simulink model "Citation_2015a"  (R2015a)
settings: Solver=ode5  StartTime=0.0  StopTime=inf  FixedStep=0.01  RelTol=1e-3
InitFcn:
  | initcit
values from neighbouring files (symbols this model uses):
  aeroinit = [dp_ini;inicoef('CX0');inicoef('CXa');inicoef('CXa2');inicoef('CXq')     ;inicoef('CXde');inicoef('CY0');inicoef('CYB');inicoef('CYp');inicoef('CYr')     ;inicoef('CYda');inicoef('CYdr');inicoef('CZ0');inicoef('CZa');inicoef('CZq')     ;inicoef('CZde');inicoef('Cl0');inicoef('ClB');inicoef('Clp');inicoef('Clr')     ;inicoef('Clda');inicoef('Cldr');inicoef('Cm0');inicoef('Cma');inicoef('Cmq')     ; ...(+113 chars)    [initcit.m]
  Clda_thresh = 3.410e-2/2    (= 0.01705)    [initcit.m]
  h_l_old = zeros(6,sample_size)    [initcit.m]
  h_m_old = zeros(4,sample_size)    [initcit.m]
  h_n_old = zeros(6,sample_size)    [initcit.m]
  h_X_old = zeros(5,sample_size)    [initcit.m]
  h_Y_old = zeros(6,sample_size)    [initcit.m]
  h_Z_old = zeros(4,sample_size)    [initcit.m]
  I = [massinit(5),0, -massinit(8);0, massinit(6),0;-massinit(8),0, massinit(7)]    [initcit.m]
  p_l = [inicoef('Cl0');inicoef('ClB');inicoef('Clp');inicoef('Clr')     ;inicoef('Clda');inicoef('Cldr')].*ones(6,sample_size)    [initcit.m]
  p_m = [inicoef('Cm0');inicoef('Cma');inicoef('Cmq')     ;inicoef('Cmde')].*ones(4,sample_size)    [initcit.m]
  p_n = [inicoef('Cn0');inicoef('CnB');inicoef('Cnp');inicoef('Cnr')     ;inicoef('Cnda');inicoef('Cndr')].*ones(6,sample_size)    [initcit.m]
  p_X = [inicoef('CX0');inicoef('CXa');inicoef('CXa2');inicoef('CXq')     ;inicoef('CXde')].*ones(5,sample_size)    [initcit.m]
  p_Y = [inicoef('CY0');inicoef('CYB');inicoef('CYp');inicoef('CYr')     ;inicoef('CYda');inicoef('CYdr')].*ones(6,sample_size)    [initcit.m]
  p_Z = [inicoef('CZ0');inicoef('CZa');inicoef('CZq')     ;inicoef('CZde')].*ones(4,sample_size)    [initcit.m]
  Pcov_l = 10000*eye(6)    [initcit.m]
  Pcov_m = 10000*eye(4)    [initcit.m]
  Pcov_n = 10000*eye(6)    [initcit.m]
  Pcov_X = 10000*eye(5)    [initcit.m]
  Pcov_Y = 10000*eye(6)    [initcit.m]
  Pcov_Z = 10000*eye(4)    [initcit.m]
  replay = 0    [initcit.m]
  T0 = 288.15    [rho_test.m]
  timeend = inputsim.data{1}.Values.Time(end)    [initcit.m]
  Vw915 = 0    [initcit.m]
  winddir = 45*(pi/180)    (= 0.785398163397)    [initcit.m]
  x0 = []    [cessnac550_3d_sfnc.m]    (also in sfunxyauto.m)
  y_l = zeros(1,sample_size)    [initcit.m]
  y_l_est_old = zeros(size(y_l))    [initcit.m]
  y_m = zeros(1,sample_size)    [initcit.m]
  y_m_est_old = zeros(size(y_m))    [initcit.m]
  y_n = zeros(1,sample_size)    [initcit.m]
  y_n_est_old = zeros(size(y_n))    [initcit.m]
  y_X = zeros(1,sample_size)    [initcit.m]
  y_X_est_old = zeros(size(y_X))    [initcit.m]
  y_Y = zeros(1,sample_size)    [initcit.m]
  y_Y_est_old = zeros(size(y_Y))    [initcit.m]
  y_Z = zeros(1,sample_size)    [initcit.m]
  y_Z_est_old = zeros(size(y_Z))    [initcit.m]
undefined symbols (not defined in the file or in its folder): chord, cv1, cv2, cv3, cv4, deltagmax1, deltagmax2, deltagmax3, deltagmax4, Deng, ealphag, ealphas, g0, hDME, hGS, kt1, kt2, kt3, lh, massinit, matbuaf, matdaf, matdam, matdbbf, matdeaf, matdgaf, matdqaf, matduaf, matdwaw, matedhr, mateif, matelhr, matemhr, matemv1, matemv2, matemve, matetam, mateuaf, matfaaf, matfaxl, matff, matibaf, matibmh, matipaf, matipmh, matiraf, matiuaf, matiwaf, matlaf, matlam, matleaf, matleam, matlgaf, matlqaf, matluaf, matmaaf, matmaam, matmaf, matmam, matmbbf ... (+74)
undefined symbols (not defined in the file): matibb
libraries: simulink x13, templibrary x6, vrlib x1
(part 2 of 7)

== system Citation_2015a/Aerodynamic Parameter Estimation/alternative failure monitor system ==
  note: this failure monitoring systems looks at the parameter related to the estimated delta_a directly. E.g. Clda
  In2 : Inport
  In3 : Inport  Port=2
  Abs : Abs
  Auto_correlation : Subsystem
  Constant : Constant  Value=Clda_thresh*2
  Constant4 : Constant
  Constant5 : Constant  Value=0
  Demux : Demux  Commented=on  Outputs=2
  Detect Change : simulink/Logic and Bit Operations/Detect Change  vinit=0  OutDataTypeStr=boolean
  Display : Display  Commented=on
  Failure Monitor : TimeScope  Commented=on  DefaultConfigurationName=spbscopes.TimeScopeBlockCfg  NumInputPorts=3
  Gain : Gain  Gain=0.5
  Memory : Memory
  Selector : Selector  NumberOfDimensions=2  InputPortWidth=1  IndexOptions=Index vector (dialog),Index vector (dialog)  Indices=[5],[1:50]  OutputSizes=1,1
  Send diagnostic message : Subsystem  Commented=on  TreatAsAtomicUnit=on
  Slider : Subsystem  Description=Replaced Block  mask(Replaced Block){}
      mask help: This block has been replaced with an empty subsystem because it used functionality that is unavailable in Simulink R2015a.
      mask Display: fprintf('Replaced: %s\n','Dashboard Widget')
  Sum : Sum  Inputs=|+-
  Switch : Switch  Criteria=u2 > Threshold  Threshold=Clda_thresh
  Variance : TimeScope  Commented=on  DefaultConfigurationName=spbscopes.TimeScopeBlockCfg  NumInputPorts=3
  auto corr : TimeScope  Commented=on  DefaultConfigurationName=spbscopes.TimeScopeBlockCfg  NumInputPorts=2
  moving average square : MATLAB Function  TreatAsAtomicUnit=on
      settings: PermitHierarchicalResolution=ParametersOnly
  variance : Subsystem  Commented=on
  Out1 : Outport
  wires:
  In3/1 -> Auto_correlation/2(kgap)
  Selector/1 -> Auto_correlation/1(delta_window), moving average square/1(delta)
  moving average square/1(av) -> Sum/1, Failure Monitor/3  "Alt Moving square average"
  variance/2(sigma_avg) -> Demux/1
  Sum/1 -> Abs/1
  Constant/1 -> Gain/1, Sum/2
  Demux/2 -> Variance/3
  variance/1(variance) -> Variance/1
  Demux/1 -> Variance/2
  In2/1 -> Selector/1
  Constant5/1 -> Switch/3
  Constant4/1 -> Switch/1
  Switch/1 -> Failure Monitor/1, Display/1, Memory/1  "alt failure detected"
  Auto_correlation/1(PI_kgap) -> auto corr/1
  Auto_correlation/2(PI_kgap_avg) -> auto corr/2
  Memory/1 -> Send diagnostic message/Trigger, Send diagnostic message/1(In1), Detect Change/1
  Gain/1 -> Failure Monitor/2  "alt threshold"
  Detect Change/1 -> Out1/1
  Abs/1 -> Switch/2

== system Citation_2015a/Aerodynamic Parameter Estimation/get_h_vectors ==
  input : Inport
  model output : Inport  Port=2
  1 : Terminator
  6 : Terminator
  Constant : Constant
  Constant1 : Constant  Value=chord
  Constant2 : Constant  Value=span
  Demux4 : Demux  Outputs=[1 1 1 1 1 1 31]
  Demux5 : Demux  Outputs=[1 1 1 7]
  Divide : Product  Inputs=*/
  Divide1 : Product  Inputs=*/
  Divide2 : Product  Inputs=*/
  Gain : Gain  Gain=2
  Multiply : Product
  Multiply1 : Product
  Mux : Mux  Inputs=6
  Mux1 : Mux  Inputs=5
  Mux2 : Mux
  Mux3 : Mux  Inputs=6
  Product : Product
  Product1 : Product
  hk : Outport
  wires:
  Demux5/2 -> Mux/5  "da"
  Demux4/6 -> Mux/2  "beta"
  Demux4/5 -> Mux1/2, Product/2, Mux2/2, Product/1  "alpha"
  Constant/1 -> Mux1/1, Mux/1, Mux2/1
  Demux4/3 -> Multiply1/1  "r"
  Demux5/4 -> 6/1
  Demux4/2 -> Product1/1  "q"
  Demux4/1 -> Multiply/2  "p"
  Demux4/4 -> Gain/1, Divide/2  "vtas"
  Constant1/1 -> Product1/2
  Product1/1 -> Divide/1
  Divide/1 -> Mux2/3, Mux1/4  "qc/V"
  model output/1 -> Demux4/1
  Demux5/1 -> Mux2/4, Mux1/5  "de"
  Product/1 -> Mux1/3
  Demux5/3 -> Mux/6  "dr"
  input/1 -> Demux5/1
  Mux1/1 -> Mux3/1  "hk_CX"
  Mux2/1 -> Mux3/3, Mux3/5  "hk_CZ & hk_Cm"
  Demux4/7 -> 1/1
  Constant2/1 -> Multiply1/2, Multiply/1
  Multiply/1 -> Divide1/1
  Gain/1 -> Divide2/2, Divide1/2
  Divide1/1 -> Mux/3  "pb/2V"
  Multiply1/1 -> Divide2/1
  Divide2/1 -> Mux/4  "rb/2V"
  Mux/1 -> Mux3/2, Mux3/6, Mux3/4
  Mux3/1 -> hk/1

== system Citation_2015a/Cessna Citation 500/Actuators ==
  note: Failure will not be visible here
  note: de
      | da
      | dr
      | dte
      | dta
      | dtr
      | df
      | gear
      | pla1
      | pla2
  note: de
      | da
      | dr
      | dte
      | dta
      | dtr
      | df
      | gear
      | pla1
      | pla2
  In : Inport
  "failure toggle " : Inport  Port=2
  Demux : Demux  Outputs=10
  Gain : Gain  Gain=0.5
  Mux : Mux  Inputs=10
  Mux2 : Mux  Inputs=10
  Subsystem : Subsystem  Commented=on
  Sum : Sum  Inputs=|++
  Switch : Switch  Criteria=u2 > Threshold
  Time Scope : TimeScope  Commented=on  DefaultConfigurationName=spbscopes.TimeScopeBlockCfg
  "aileron failure offset (deg) " : Constant  Value=16
  da : Subsystem
  da limits : Saturate  UpperLimit=0.65  LowerLimit=-0.65
  da limits1 : Saturate  UpperLimit=0.65  LowerLimit=-0.65
  da limits2 : Saturate  UpperLimit=0.65  LowerLimit=-0.65
  da2 : Subsystem
  de : Subsystem
  de limits : Saturate  UpperLimit=0.26  LowerLimit=-0.35
  deg2rad : Gain  Gain=pi/180
  dr : Subsystem
  dr limits : Saturate  UpperLimit=0.38  LowerLimit=-0.38
  flaps : Subsystem
  gear : Subsystem
  Actuator_True : Outport
  Actuator_pred : Outport  Port=2
  wires:
  In/1 -> Demux/1
  Mux/1 -> Actuator_True/1
  Demux/1 -> de/1(In)
  Demux/2 -> Switch/3, da limits1/1, da/1(In)  "da desired"
  Demux/3 -> dr/1(In)
  de/1(Out) -> de limits/1
  da/1(Out) -> da limits/1
  dr/1(Out) -> dr limits/1
  dr limits/1 -> Mux2/3, Mux/3
  de limits/1 -> Mux/1, Mux2/1
  Demux/8 -> gear/1(In)
  Demux/7 -> flaps/1(In)
  Demux/9 -> Mux2/9, Mux/9
  Demux/10 -> Mux2/10, Mux/10
  flaps/1(Out) -> Mux2/7, Mux/7
  gear/1(Out) -> Mux/8, Mux2/8
  Demux/4 -> Mux2/4, Mux/4
  Demux/5 -> Mux2/5, Mux/5
  Demux/6 -> Mux2/6, Mux/6
  da limits/1 -> Mux2/2
  "aileron failure offset (deg) "/1 -> deg2rad/1
  deg2rad/1 -> Sum/1  "da offset"
  Gain/1 -> Sum/2
  Switch/1 -> da2/1(In)
  Mux2/1 -> Actuator_pred/1
  "failure toggle "/1 -> Switch/2
  Sum/1 -> Switch/1
  da limits2/1 -> Time Scope/1, Mux/2
  da2/1(Out) -> da limits2/1
  da limits1/1 -> Gain/1

== system Citation_2015a/Cessna Citation 500/Citation model DASMAT ==
  ua : Inport
  ut : Inport  Port=2
  Environment : Inport  Port=3
  AIRCRAFT MODEL : Subsystem
  Mux1 : Mux  Inputs=[8 2 8 12 8]
  Terminator_{16..19} (4 alike) : Terminator
  massinit : Constant  Value=massinit
  x : Outport
  xdot : Outport  Port=2
  yair : Outport  Port=3
  yacc : Outport  Port=4
  yfp : Outport  Port=5
  ypp : Outport  Port=6
  wires:
  AIRCRAFT MODEL/13(FMt) -> Terminator_19/1
  Mux1/1 -> yair/1
  AIRCRAFT MODEL/12(FMag) -> Terminator_17/1
  AIRCRAFT MODEL/11(FMa) -> Terminator_18/1
  AIRCRAFT MODEL/7(gust) -> Mux1/5
  AIRCRAFT MODEL/6(wind) -> Mux1/4
  AIRCRAFT MODEL/5(yad2) -> Mux1/3
  AIRCRAFT MODEL/4(yad1) -> Mux1/2
  AIRCRAFT MODEL/3(yatm) -> Mux1/1
  AIRCRAFT MODEL/2(xdot) -> xdot/1
  AIRCRAFT MODEL/1(x) -> x/1
  AIRCRAFT MODEL/10(ys) -> Terminator_16/1
  AIRCRAFT MODEL/9(yfp) -> yfp/1
  AIRCRAFT MODEL/8(yacc) -> yacc/1
  massinit/1 -> AIRCRAFT MODEL/3(massinit)
  ut/1 -> AIRCRAFT MODEL/2(ut)
  ua/1 -> AIRCRAFT MODEL/1(ua)
  Environment/1 -> AIRCRAFT MODEL/4(Environment)
  AIRCRAFT MODEL/14(ypp) -> ypp/1

== system Citation_2015a/Cessna Citation 500/trim conditions ==
  PLA1/Tx1 : Constant  Value=ut0(1)
  PLA2/Tx2 : Constant  Value=ut0(2)
  control inputs : Mux  Inputs=8
      settings: DisplayOption=signals
  deltaa : Constant  Value=u0(2)
  deltae : Constant  Value=u0(1)
  deltaf : Constant  Value=u0(7)
  deltar : Constant  Value=u0(3)
  deltata : Constant  Value=u0(5)
  deltate : Constant  Value=u0(4)
  deltatr : Constant  Value=u0(6)
  engine inputs : Mux  Inputs=2
      settings: DisplayOption=signals
  lgsw : Constant  Value=u0(8)
  ua : Outport
  ut : Outport  Port=2
  wires:
  deltaf/1 -> control inputs/7  "df"
  engine inputs/1 -> ut/1
  deltatr/1 -> control inputs/6  "dtr"
  deltata/1 -> control inputs/5  "dta"
  control inputs/1 -> ua/1
  PLA1/Tx1/1 -> engine inputs/1  "pla1"
  PLA2/Tx2/1 -> engine inputs/2  "pla2"
  deltae/1 -> control inputs/1  "de"
  deltaa/1 -> control inputs/2  "da"
  deltar/1 -> control inputs/3  "dr"
  deltate/1 -> control inputs/4  "dte"
  lgsw/1 -> control inputs/8  "lg"

== system Citation_2015a/Controllers/ANDI rotational rate controller ==
  note: To A/C
  note: u=b^-1(v-a)
  note: p
      | q
      | r
      | vtas
      | alpha
      | beta
      | phi
      | theta
      | psi
      | he
      | xe
      | ye
  note: de
      | da
      | dr
      | dte
      | dta
      | dtr
      | df
      | gear
      | pla1
      | pla2
  note: [1]
  note: Cl0
      | ClB
      | Clp
      | Clr
      | Clda
      | Cldr
  note: dynamic pressure
  note: CZ0
      | CZa
      | CZq
      | CZde
  note: CY0
      | CYB
      | CYp
      | CYr
      | CYda
      | CYdr
  note: Cn0
      | CnB
      | Cnp
      | Cnr
      | Cnda
      | Cndr
  note: CX0
      | CXa
      | CXa^2
      | CXq
      | CXde
  note: Cm0
      | Cma
      | Cmq
      | Cmde
  note: [23:26]
  note: [13:16]
  note: [27:32]
  note: [17:22]
  note: [7:12]
  note: [2:6]
  note: Aerodata Description
  note: de
      | da
      | dr
      | dte
      | dta
      | dtr
      | df
      | gear
      | pla1
      | pla2
  note: From A/C
  inputs : Inport
  A/C state : Inport  Port=2
  aero data : Inport  Port=3
  int reset : Inport  Port=4
  Demux : Demux  Outputs=[1 1 1 7]
  Demux1 : Demux  Outputs=[3 9]
  Demux2 : Demux  Outputs=3
  Linear Controller : Subsystem
  Memory : Memory  X0=eye(3)
  Mux : Mux  Inputs=3
  Mux1 : Mux
  Sum : Sum  Inputs=+-
  Sum1 : Sum  Inputs=|+-
  Terminator1 : Terminator
  a : MATLAB Function  TreatAsAtomicUnit=on
      settings: PermitHierarchicalResolution=ParametersOnly
  b^-1 : MATLAB Function  TreatAsAtomicUnit=on
      settings: PermitHierarchicalResolution=ParametersOnly
  da limits : Saturate  UpperLimit=0.65  LowerLimit=-0.65
  de limits : Saturate  UpperLimit=0.26  LowerLimit=-0.35
  dr limits : Saturate  UpperLimit=0.38  LowerLimit=-0.38
  control input : Outport
  wires:
  inputs/1 -> Demux/1
  Demux1/2 -> Terminator1/1
  Demux1/1 -> Sum/2  "p q r"
  A/C state/1 -> a/2(state), Demux1/1
  Mux1/1 -> control input/1
  aero data/1 -> a/1(aerodat), b^-1/2(aerodat)
  b^-1/2(mat_old) -> Memory/1
  Memory/1 -> b^-1/3("mat_old ")
  Demux/4 -> [RC]
  [RC] -> Mux1/4
  Demux2/2 -> de limits/1  "de"
  Demux2/1 -> da limits/1  "da"
  Demux2/3 -> dr limits/1  "dr"
  a/1(y) -> Sum1/2
  Linear Controller/1(v) -> Sum1/1  "vp vq vr"
  b^-1/1(delta) -> Demux2/1  "da de dr"
  Mux/1 -> Sum/1  "pref qref rref"
  de limits/1 -> Mux1/1  "de"
  da limits/1 -> Mux1/2
  dr limits/1 -> Mux1/3  "dr"
  int reset/1 -> Linear Controller/2(int reset)
  Sum/1 -> Linear Controller/1(e_omega)
  Sum1/1 -> b^-1/1(ve)
  Demux/1 -> Mux/1
  Demux/2 -> Mux/2
  Demux/3 -> Mux/3

== system Citation_2015a/Controllers/Classical rotational rate control ==
  note: de
      | da
      | dr
      | dte
      | dta
      | dtr
      | df
      | gear
      | pla1
      | pla2
  note: p
      | q
      | r
      | vtas
      | alpha
      | beta
      | phi
      | theta
      | psi
      | he
      | xe
      | ye
  inputs : Inport
  state : Inport  Port=2
  int reset : Inport  Port=3
  Demux : Demux  Outputs=[1 1 1 7]
  Demux1 : Demux  Outputs=[1 1 1 2 1 6]
  Display1 : Display
  Gain14 : Gain
  Mux : Mux
  PID Controller : simulink/Continuous/PID Controller  Controller=PID  TimeDomain=Continuous-time  SampleTime=-1  IntegratorMethod=Forward Euler  FilterMethod=Forward Euler  Form=Parallel  UseFilter=on  ControllerParametersSource=internal  P=-2  I=-0.1  D=0  N=1  InitialConditionSource=internal  InitialConditionForIntegrator=0  InitialConditionForFilter=0  ExternalReset=rising  LimitOutput=off  UpperSaturationLimit=inf  LowerSaturationLimit=-inf  LinearizeAsGain=on  AntiWindupMode=none  Kb=1  TrackingMode=off  Kt=1  PParamMin=[]  PParamMax=[]  IParamMin=[]  IParamMax=[]  DParamMin=[]  DParamMax=[]  NParamMin=[]  NParamMax=[]  KbParamMin=[]  KbParamMax=[]  KtParamMin=[]  KtParamMax=[]  POutMin=[]  POutMax=[]  IOutMin=[]  IOutMax=[]  DOutMin=[]  DOutMax=[]  NOutMin=[]  NOutMax=[]  KbOutMin=[]  KbOutMax=[]  KtOutMin=[]  KtOutMax=[]  IntegratorOutMin=[]  IntegratorOutMax=[]  FilterOutMin=[]  FilterOutMax=[]  SumOutMin=[]  SumOutMax=[]  SumI1OutMin=[]  SumI1OutMax=[]  SumI2OutMin=[]  SumI2OutMax=[]  SumI3OutMin=[]  SumI3OutMax=[]  SumDOutMin=[]  SumDOutMax=[]  SaturationOutMin=[]  SaturationOutMax=[]  IntegratorContinuousStateAttributes=''  IntegratorStateMustResolveToSignalObject=off  IntegratorRTWStateStorageClass=Auto  FilterContinuousStateAttributes=''  FilterStateMustResolveToSignalObject=off  FilterRTWStateStorageClass=Auto  DifferentiatorICPrevScaledInput=0  DifferentiatorOutMin=[]  DifferentiatorOutMax=[]
  PID Controller1 : simulink/Continuous/PID Controller  Controller=PID  TimeDomain=Continuous-time  SampleTime=-1  IntegratorMethod=Forward Euler  FilterMethod=Forward Euler  Form=Parallel  UseFilter=on  ControllerParametersSource=internal  P=-1  I=-0.5  D=0  N=100  InitialConditionSource=internal  InitialConditionForIntegrator=0  InitialConditionForFilter=0  ExternalReset=rising  LimitOutput=off  UpperSaturationLimit=inf  LowerSaturationLimit=-inf  LinearizeAsGain=on  AntiWindupMode=none  Kb=1  TrackingMode=off  Kt=1  PParamMin=[]  PParamMax=[]  IParamMin=[]  IParamMax=[]  DParamMin=[]  DParamMax=[]  NParamMin=[]  NParamMax=[]  KbParamMin=[]  KbParamMax=[]  KtParamMin=[]  KtParamMax=[]  POutMin=[]  POutMax=[]  IOutMin=[]  IOutMax=[]  DOutMin=[]  DOutMax=[]  NOutMin=[]  NOutMax=[]  KbOutMin=[]  KbOutMax=[]  KtOutMin=[]  KtOutMax=[]  IntegratorOutMin=[]  IntegratorOutMax=[]  FilterOutMin=[]  FilterOutMax=[]  SumOutMin=[]  SumOutMax=[]  SumI1OutMin=[]  SumI1OutMax=[]  SumI2OutMin=[]  SumI2OutMax=[]  SumI3OutMin=[]  SumI3OutMax=[]  SumDOutMin=[]  SumDOutMax=[]  SaturationOutMin=[]  SaturationOutMax=[]  IntegratorContinuousStateAttributes=''  IntegratorStateMustResolveToSignalObject=off  IntegratorRTWStateStorageClass=Auto  FilterContinuousStateAttributes=''  FilterStateMustResolveToSignalObject=off  FilterRTWStateStorageClass=Auto  DifferentiatorICPrevScaledInput=0  DifferentiatorOutMin=[]  DifferentiatorOutMax=[]
  PID Controller2 : simulink/Continuous/PID Controller  Controller=PID  TimeDomain=Continuous-time  SampleTime=-1  IntegratorMethod=Forward Euler  FilterMethod=Forward Euler  Form=Parallel  UseFilter=on  ControllerParametersSource=internal  P=-2  I=-0.1  D=0  N=100  InitialConditionSource=internal  InitialConditionForIntegrator=0  InitialConditionForFilter=0  ExternalReset=rising  LimitOutput=off  UpperSaturationLimit=inf  LowerSaturationLimit=-inf  LinearizeAsGain=on  AntiWindupMode=none  Kb=1  TrackingMode=off  Kt=1  PParamMin=[]  PParamMax=[]  IParamMin=[]  IParamMax=[]  DParamMin=[]  DParamMax=[]  NParamMin=[]  NParamMax=[]  KbParamMin=[]  KbParamMax=[]  KtParamMin=[]  KtParamMax=[]  POutMin=[]  POutMax=[]  IOutMin=[]  IOutMax=[]  DOutMin=[]  DOutMax=[]  NOutMin=[]  NOutMax=[]  KbOutMin=[]  KbOutMax=[]  KtOutMin=[]  KtOutMax=[]  IntegratorOutMin=[]  IntegratorOutMax=[]  FilterOutMin=[]  FilterOutMax=[]  SumOutMin=[]  SumOutMax=[]  SumI1OutMin=[]  SumI1OutMax=[]  SumI2OutMin=[]  SumI2OutMax=[]  SumI3OutMin=[]  SumI3OutMax=[]  SumDOutMin=[]  SumDOutMax=[]  SaturationOutMin=[]  SaturationOutMax=[]  IntegratorContinuousStateAttributes=''  IntegratorStateMustResolveToSignalObject=off  IntegratorRTWStateStorageClass=Auto  FilterContinuousStateAttributes=''  FilterStateMustResolveToSignalObject=off  FilterRTWStateStorageClass=Auto  DifferentiatorICPrevScaledInput=0  DifferentiatorOutMin=[]  DifferentiatorOutMax=[]
  Sum : Sum  Inputs=|+-
  Sum1 : Sum  Inputs=|+-
  Sum2 : Sum  Inputs=|+-
  Terminator : Terminator
  Terminator1 : Terminator
  Time Scope : TimeScope  Commented=on  DefaultConfigurationName=spbscopes.TimeScopeBlockCfg  NumInputPorts=2
  beta : TimeScope  Commented=on  DefaultConfigurationName=spbscopes.TimeScopeBlockCfg  NumInputPorts=3
  q : TimeScope  Commented=on  DefaultConfigurationName=spbscopes.TimeScopeBlockCfg  NumInputPorts=3
  control inputs : Outport
  wires:
  inputs/1 -> Demux/1
  Demux/2 -> q/1, Sum/1  "qref"
  Mux/1 -> Display1/1, control inputs/1
  state/1 -> Demux1/1
  Demux1/4 -> Terminator/1
  Sum/1 -> q/3, PID Controller2/1  "qe"
  Sum1/1 -> PID Controller1/1
  Demux/1 -> Time Scope/1, Sum1/1  "pref"
  Demux1/1 -> Time Scope/2, Sum1/2  "p"
  Demux1/2 -> q/2, Sum/2  "q"
  Demux1/3 -> Sum2/2  "r"
  Sum2/1 -> PID Controller/1
  PID Controller2/1 -> Mux/1
  PID Controller1/1 -> Mux/2
  PID Controller/1 -> Mux/3
  Demux/3 -> beta/3, Gain14/1  "rref"
  Demux1/6 -> Terminator1/1
  Demux1/5 -> beta/2  "beta"
  Gain14/1 -> Sum2/1
  int reset/1 -> PID Controller/2, PID Controller1/2, PID Controller2/2
  Demux/4 -> Mux/4

== system Citation_2015a/Controllers/Default Actuator Control ==
  state : Inport
  inputs : Inport  Port=2
  A/T 1 : Gain  Gain=[1 1 1 1 1 1 1 1 1 1]  SaturateOnIntegerOverflow=on  OutDataTypeStr=Inherit: Same as input  ParamDataTypeStr=Inherit: Same as input
  A/T disabled1 : Gain  Gain=0  SaturateOnIntegerOverflow=on  OutDataTypeStr=Inherit: Same as input  ParamDataTypeStr=Inherit: Same as input
  Gain1 : Gain
  Yaw damper1 : Subsystem
  add controller outputs to pilot inputs1 : Sum  Inputs=|+|+|+|  SaturateOnIntegerOverflow=on
  auto throttle1 : Subsystem
  control inputs : Outport
  wires:
  add controller outputs to pilot inputs1/1 -> control inputs/1
  auto throttle1/1(controller output) -> A/T disabled1/1
  A/T disabled1/1 -> add controller outputs to pilot inputs1/2
  Gain1/1 -> add controller outputs to pilot inputs1/1
  A/T 1/1 -> add controller outputs to pilot inputs1/3
  Yaw damper1/1(controller output) -> Gain1/1
  state/1 -> auto throttle1/1(state), Yaw damper1/1(state)
  inputs/1 -> A/T 1/1, Yaw damper1/2(inputs), auto throttle1/2(inputs)

== system Citation_2015a/Controllers/Generate Integral reset pulse ==
  mode toggle : Inport
  fail detect : Inport  Port=2
  manual_reset : Inport  Port=3
  Constant2 : Constant
  Constant4 : Constant  Value=0
  Detect Change : simulink/Logic and Bit Operations/Detect Change  vinit=0  OutDataTypeStr=boolean
  Detect Change1 : simulink/Logic and Bit Operations/Detect Change  vinit=0  OutDataTypeStr=boolean
  Sum : Sum  Inputs=|+|+|+|
  Switch : Switch  Criteria=u2 > Threshold
  reset_pulse : Outport
  wires:
  Switch/1 -> reset_pulse/1
  Sum/1 -> Switch/2
  fail detect/1 -> Sum/2  "fail detected"
  mode toggle/1 -> Detect Change/1
  Detect Change/1 -> Sum/1  "control mode switched"
  Constant4/1 -> Switch/3
  Constant2/1 -> Switch/1
  manual_reset/1 -> Detect Change1/1
  Detect Change1/1 -> Sum/3  "manual"

== system Citation_2015a/Controllers/INDI rotational rate controller ==
  note: Actuator Dynamics
  note: The actuator dynamics are replicated for convenience. Otherwise it should have been brought out of the citation mask
  note: note: INDI uses a constant aerodynamic model.
      | Here only the dynamic pressures from the airdata signal is used
  note: pdot
      | qdot
      | rdot
      | VTASdot
      | hedot
  Inputs : Inport
  state : Inport  Port=2
  int reset : Inport  Port=3
  xdot : Inport  Port=4
  airdata : Inport  Port=5
  Demux : Demux  Outputs=[3 7]
  Demux1 : Demux  Outputs=[3 9]
  Demux2 : Demux  Outputs=[3 2]
  Demux3 : Demux  Outputs=[1 31]
  Demux5 : Demux  Outputs=3
  Demux6 : Demux  Commented=on  Outputs=3
  Demux7 : Demux  Commented=on  Outputs=[1 2]
  INDI : MATLAB Function  TreatAsAtomicUnit=on
      settings: PermitHierarchicalResolution=ParametersOnly
  INDI  pqr errors : TimeScope  Commented=on  DefaultConfigurationName=spbscopes.TimeScopeBlockCfg  NumInputPorts=3
  Linear Controller : Subsystem
  Mux : Mux  Inputs=2
  Mux1 : Mux  Inputs=3
  Sum : Sum  Inputs=|+-
  Sum1 : Sum  Inputs=|+-
  Terminator : Terminator
  Terminator1 : Terminator
  Terminator2 : Terminator
  Terminator3 : Terminator  Commented=on
  Time Scope2 : TimeScope  Commented=on  DefaultConfigurationName=spbscopes.TimeScopeBlockCfg  NumInputPorts=2
  Transfer Fcn : TransferFcn  Denominator=[0.1 1]
  Transfer Fcn1 : TransferFcn  Denominator=[0.1 1]
  Transfer Fcn2 : TransferFcn  Denominator=[0.1 1]
  da limits : Saturate  UpperLimit=0.65  LowerLimit=-0.65
  de limits : Saturate  UpperLimit=0.26  LowerLimit=-0.35
  dr limits : Saturate  UpperLimit=0.38  LowerLimit=-0.38
  Out1 : Outport
  wires:
  int reset/1 -> Linear Controller/2(int reset)
  Inputs/1 -> Demux/1
  state/1 -> Demux1/1
  Demux1/2 -> Terminator/1
  Demux/1 -> Sum/1
  Demux1/1 -> Sum/2
  Sum/1 -> Linear Controller/1(e_omega)
  Linear Controller/1(v) -> Sum1/1  "vp vq vr"
  xdot/1 -> Demux2/1
  Demux2/2 -> Terminator1/1
  Demux2/1 -> Sum1/2
  airdata/1 -> Demux3/1
  Demux3/2 -> Terminator2/1
  Demux3/1 -> INDI/1(dp)  "dynamic pressure (0.5*rho*V^2*S)"
  Sum1/1 -> INDI/2(e_omegadot)
  INDI/1(control_input) -> Demux5/1, Mux/1  "de da dr"
  Demux/2 -> Mux/2
  Mux/1 -> Out1/1
  de limits/1 -> Mux1/1
  da limits/1 -> Mux1/2
  dr limits/1 -> Mux1/3
  Demux5/2 -> Transfer Fcn/1
  Transfer Fcn1/1 -> de limits/1
  Demux5/1 -> Transfer Fcn1/1
  Demux5/3 -> Transfer Fcn2/1
  Transfer Fcn2/1 -> dr limits/1
  Transfer Fcn/1 -> da limits/1
  Demux6/1 -> INDI  pqr errors/1  "p"
  Demux6/2 -> INDI  pqr errors/2  "q"
  Demux6/3 -> INDI  pqr errors/3  "r"
  Demux7/2 -> Terminator3/1
  Demux7/1 -> Time Scope2/1  "pref"
  Mux1/1 -> INDI/3("control_input ")

== system Citation_2015a/Controllers/Input to omega_ref (Beta feedback included) ==
  note: p
      | q
      | r
  note: And scale to max angular rates
  note: 1st order filters
  note: normalize inputs back from deflection values
  Input : Inport
  state : Inport  Port=2
  Demux : Demux  Outputs=[5 1 6]
  Demux1 : Demux  Outputs=[1 1 1 7]
  Gain : Gain  Gain=-1
  Gain1 : Gain  Gain=-1  SaturateOnIntegerOverflow=on  OutDataTypeStr=Inherit: Same as input  ParamDataTypeStr=Inherit: Same as input
  Gain10 : Gain  Gain=180/pi  SaturateOnIntegerOverflow=on  OutDataTypeStr=Inherit: Same as input  ParamDataTypeStr=Inherit: Same as input
  Gain11 : Gain  Gain=180/pi  SaturateOnIntegerOverflow=on  OutDataTypeStr=Inherit: Same as input  ParamDataTypeStr=Inherit: Same as input
  Gain12 : Gain  Gain=pi/2  SaturateOnIntegerOverflow=on  OutDataTypeStr=Inherit: Same as input  ParamDataTypeStr=Inherit: Same as input
  Gain13 : Gain  Gain=-1
  Gain2 : Gain  Gain=-1  SaturateOnIntegerOverflow=on  OutDataTypeStr=Inherit: Same as input  ParamDataTypeStr=Inherit: Same as input
  Gain3 : Gain  Gain=5  SaturateOnIntegerOverflow=on  OutDataTypeStr=Inherit: Same as input  ParamDataTypeStr=Inherit: Same as input
  Gain4 : Gain  Gain=-1  SaturateOnIntegerOverflow=on  OutDataTypeStr=Inherit: Same as input  ParamDataTypeStr=Inherit: Same as input
  Gain5 : Gain  Gain=1/37.24  SaturateOnIntegerOverflow=on  OutDataTypeStr=Inherit: Same as input  ParamDataTypeStr=Inherit: Same as input
  Gain6 : Gain  Gain=1/20  SaturateOnIntegerOverflow=on  OutDataTypeStr=Inherit: Same as input  ParamDataTypeStr=Inherit: Same as input
  Gain7 : Gain  Gain=1.5  SaturateOnIntegerOverflow=on  OutDataTypeStr=Inherit: Same as input  ParamDataTypeStr=Inherit: Same as input
  Gain8 : Gain  Gain=1/22  SaturateOnIntegerOverflow=on  OutDataTypeStr=Inherit: Same as input  ParamDataTypeStr=Inherit: Same as input
  Gain9 : Gain  Gain=180/pi  SaturateOnIntegerOverflow=on  OutDataTypeStr=Inherit: Same as input  ParamDataTypeStr=Inherit: Same as input
  Mux : Mux
  Sum : Sum  Inputs=|+-
  Terminator : Terminator
  Terminator1 : Terminator
  Time Scope : TimeScope  Commented=on  DefaultConfigurationName=spbscopes.TimeScopeBlockCfg  NumInputPorts=2
  Transfer Fcn : TransferFcn  Denominator=[0.1 1]
  Transfer Fcn1 : TransferFcn  Denominator=[0.1 1]
  Transfer Fcn2 : TransferFcn  Denominator=[0.1 1]
  omega_ref : Outport
  wires:
  Gain12/1 -> Transfer Fcn2/1
  Demux1/2 -> Gain1/1
  Gain11/1 -> Gain12/1
  Gain10/1 -> Gain7/1
  Demux1/1 -> Gain2/1
  Gain8/1 -> Gain11/1
  Demux1/3 -> Gain4/1
  Gain3/1 -> Time Scope/2, Transfer Fcn1/1
  Transfer Fcn/1 -> Mux/2  "qref"
  Gain9/1 -> Gain3/1
  Gain4/1 -> Gain8/1
  Gain2/1 -> Gain6/1
  Gain6/1 -> Gain10/1
  Gain1/1 -> Gain5/1
  Gain5/1 -> Gain9/1
  Input/1 -> Demux1/1
  Transfer Fcn1/1 -> Time Scope/1, Mux/1  "pref"
  Transfer Fcn2/1 -> Gain/1  "beta ref"
  Gain/1 -> Sum/1
  Sum/1 -> Gain13/1
  Demux/1 -> Terminator1/1
  state/1 -> Demux/1
  Demux/3 -> Terminator/1
  Demux/2 -> Sum/2  "beta"
  Gain13/1 -> Mux/3
  Mux/1 -> omega_ref/1  "omegaref"
  Demux1/4 -> Mux/4
  Gain7/1 -> Transfer Fcn/1

== system Citation_2015a/Controllers/auto throttle ==
  state : Inport
  inputs : Inport  Port=2
  Gain : Gain  Gain=0.5  SaturateOnIntegerOverflow=on  OutDataTypeStr=Inherit: Same as input  ParamDataTypeStr=Inherit: Same as input
  Saturation : Saturate  UpperLimit=1.0  LowerLimit=0.0
  Sum : Sum  Inputs=+-|  SaturateOnIntegerOverflow=on
  VTAS ref (trim value) : Constant  Value=x0(4)
  VTAS sel : Selector  IndexOptions=Index vector (dialog)  Indices=[4]  OutputSizes=1
  controller output is later added to pilot input! : Sum  Inputs=|+-  SaturateOnIntegerOverflow=on
  pla1&2 : Gain  Gain=[0 0 0 0 0 0 0 0 1 1]  SaturateOnIntegerOverflow=on  OutDataTypeStr=Inherit: Same as input  ParamDataTypeStr=Inherit: Same as input
  pla1&2 as well : Gain  Gain=[0 0 0 0 0 0 0 0 1 1]  SaturateOnIntegerOverflow=on  OutDataTypeStr=Inherit: Same as input  ParamDataTypeStr=Inherit: Same as input
  controller output : Outport
  wires:
  inputs/1 -> pla1&2 as well/1
  state/1 -> VTAS sel/1
  VTAS sel/1 -> Sum/2  "VTAS"
  VTAS ref (trim value)/1 -> Sum/1
  Sum/1 -> Gain/1
  pla1&2/1 -> controller output is later added to pilot input!/1
  Gain/1 -> Saturation/1
  controller output is later added to pilot input!/1 -> controller output/1
  Saturation/1 -> pla1&2/1
  pla1&2 as well/1 -> controller output is later added to pilot input!/2

== system Citation_2015a/Flight Monitoring/3D Display ==
  roll : Inport
  pitch : Inport  Port=2
  yaw : Inport  Port=3
  Mux1 : Mux
  Position : Subsystem
  S-Function : S-Function  FunctionName=cessnac550_3d_sfnc  SFunctionDeploymentMode=off  EnableBusSupport=off
  Stop Simulation : Stop
  wires:
  roll/1 -> Mux1/1
  Position/1(Out1) -> Mux1/4
  pitch/1 -> Mux1/2
  yaw/1 -> Mux1/3
  Mux1/1 -> S-Function/1
  S-Function/1 -> Stop Simulation/1

== system Citation_2015a/Pilot/Joystick ==
  note: Set to correct ID when switching between joysticks
  Constant2 : Constant  Value=replay
  Demux : Demux  Outputs=11
  DualShock : Subsystem  Commented=on
  Joystick Input : vrlib/Joystick Input  joyid=1  adjustports=on  forcefeed=off
  Logitech 3D Pro : Subsystem
  Mux : Mux  Inputs=2
  Stop sim when replay has ended : Subsystem
  Sum : Sum  Inputs=|++
  Switch1 : Switch  Criteria=u2 > Threshold
  Terminator5 : Terminator
  load pre-recorded inputs : Subsystem
  delta elevator : Outport
  delta aileron : Outport  Port=2
  delta rudder : Outport  Port=3
  Throttle setting : Outport  Port=4
  "Failure Button " : Outport  Port=5
  NDI Button : Outport  Port=6
  Default Mode button : Outport  Port=7
  Classical rate Mode button : Outport  Port=8
  INDI mode button : Outport  Port=9
  man_int_reset : Outport  Port=10
  "Autothrottle " : Outport  Port=11
  wires:
  Joystick Input/3 -> Terminator5/1
  Joystick Input/1 -> Mux/1
  Joystick Input/2 -> Mux/2
  DualShock/1("Model Input ") -> Sum/1
  Logitech 3D Pro/1(Model Input) -> Sum/2
  Sum/1 -> Demux/1
  Demux/1 -> delta aileron/1
  Demux/2 -> delta elevator/1
  Demux/3 -> Throttle setting/1
  Demux/4 -> delta rudder/1
  Demux/5 -> "Failure Button "/1
  Demux/6 -> Classical rate Mode button/1
  Demux/7 -> INDI mode button/1
  Demux/8 -> Default Mode button/1
  Demux/9 -> NDI Button/1
  Demux/10 -> man_int_reset/1
  Demux/11 -> "Autothrottle "/1
  Mux/1 -> Switch1/3
  Switch1/1 -> Logitech 3D Pro/1("JoyStick Input ")  "joystick"
  Constant2/1 -> Switch1/2, Stop sim when replay has ended/1(In1)
  load pre-recorded inputs/1(Out1) -> Switch1/1

== system Citation_2015a/Pilot/Select new mode ==
  note: only triggered by a change
  note: default value
  In1 : Inport
  In2 : Inport  Port=2
  In3 : Inport  Port=3
  In4 : Inport  Port=4
  Constant1 : Constant  Value=4
  Detect Change : simulink/Logic and Bit Operations/Detect Change  vinit=0  OutDataTypeStr=boolean
  Mux1 : Mux
  Sum1 : Sum  Inputs=++++
  Switch1 : Switch  Criteria=u2 > Threshold
  Time Scope : TimeScope  Commented=on  DefaultConfigurationName=spbscopes.TimeScopeBlockCfg
  Triggered Subsystem : Subsystem  TreatAsAtomicUnit=on
  Out1 : Outport
  wires:
  In3/1 -> Sum1/3, Mux1/3
  Constant1/1 -> Switch1/3
  In4/1 -> Sum1/1, Mux1/1
  Mux1/1 -> Triggered Subsystem/1(triggers)
  In1/1 -> Sum1/2, Mux1/2
  In2/1 -> Sum1/4, Mux1/4
  Triggered Subsystem/1(index) -> Switch1/1, Switch1/2
  Detect Change/1 -> Triggered Subsystem/Trigger
  Sum1/1 -> Detect Change/1
  Switch1/1 -> Time Scope/1, Out1/1

== system Citation_2015a/Pilot/button2toggle 1 ==
  In1 : Inport
  Trigger : TriggerPort  PortDimensions=1
  Constant1 : Constant
  Constant2 : Constant  Value=0
  Memory : Memory  InheritSampleTime=on
  Multiply : Product
  Switch : Switch  Criteria=u2 > Threshold
  Out1 : Outport
  wires:
  Constant2/1 -> Switch/1
  Switch/1 -> Memory/1, Out1/1
  Memory/1 -> Switch/2
  Constant1/1 -> Multiply/1
  Multiply/1 -> Switch/3
  In1/1 -> Multiply/2

== system Citation_2015a/Pilot/button2toggle 2 ==
  In1 : Inport
  Trigger : TriggerPort  PortDimensions=1
  Constant1 : Constant
  Constant2 : Constant  Value=0
  Memory : Memory  InheritSampleTime=on
  Multiply : Product
  Switch : Switch  Criteria=u2 > Threshold
  Out1 : Outport
  wires:
  In1/1 -> Multiply/2
  Multiply/1 -> Switch/3
  Constant1/1 -> Multiply/1
  Memory/1 -> Switch/2
  Switch/1 -> Out1/1, Memory/1
  Constant2/1 -> Switch/1

== system Citation_2015a/Pilot/button2toggle 3 ==
  In1 : Inport
  Trigger : TriggerPort  PortDimensions=1
  Constant1 : Constant
  Constant2 : Constant  Value=0
  Memory : Memory  InheritSampleTime=on
  Multiply : Product
  Switch : Switch  Criteria=u2 > Threshold
  Out1 : Outport
  wires:
  Constant2/1 -> Switch/1
  Switch/1 -> Memory/1, Out1/1
  Memory/1 -> Switch/2
  Constant1/1 -> Multiply/1
  Multiply/1 -> Switch/3
  In1/1 -> Multiply/2

== system Citation_2015a/Pilot/button2toggle 4 ==
  In1 : Inport
  Trigger : TriggerPort  PortDimensions=1
  Constant1 : Constant
  Constant2 : Constant  Value=0
  Memory : Memory  InheritSampleTime=on
  Multiply : Product
  Switch : Switch  Criteria=u2 > Threshold
  Out1 : Outport
  wires:
  In1/1 -> Multiply/2
  Multiply/1 -> Switch/3
  Constant1/1 -> Multiply/1
  Memory/1 -> Switch/2
  Switch/1 -> Out1/1, Memory/1
  Constant2/1 -> Switch/1

== system Citation_2015a/Pilot/button2toggle 5 ==
  In1 : Inport
  Trigger : TriggerPort  PortDimensions=1
  Constant1 : Constant
  Constant2 : Constant  Value=0
  MATLAB Function : MATLAB Function  TreatAsAtomicUnit=on
      settings: PermitHierarchicalResolution=ParametersOnly
  Memory : Memory  InheritSampleTime=on
  Multiply : Product
  Switch : Switch  Criteria=u2 > Threshold
  Out1 : Outport
  wires:
  Constant2/1 -> Switch/1
  Switch/1 -> Memory/1, MATLAB Function/1(u), Out1/1
  Memory/1 -> Switch/2
  Constant1/1 -> Multiply/1
  Multiply/1 -> Switch/3
  In1/1 -> Multiply/2

== system Citation_2015a/Pilot/button2toggle 6 ==
  In1 : Inport
  Trigger : TriggerPort  PortDimensions=1
  Constant1 : Constant
  Constant2 : Constant  Value=0
  MATLAB Function : MATLAB Function  TreatAsAtomicUnit=on
      settings: PermitHierarchicalResolution=ParametersOnly
  Memory : Memory  InheritSampleTime=on
  Multiply : Product
  Switch : Switch  Criteria=u2 > Threshold
  Out1 : Outport
  wires:
  Constant2/1 -> Switch/1
  Switch/1 -> Memory/1, Out1/1
  Memory/1 -> Switch/2
  Constant1/1 -> Multiply/1
  Multiply/1 -> Switch/3
  In1/1 -> Multiply/2

== system Citation_2015a/Pilot/button2toggle 7 ==
  In1 : Inport
  Trigger : TriggerPort  PortDimensions=1
  Constant1 : Constant
  Constant2 : Constant  Value=0
  MATLAB Function : MATLAB Function  TreatAsAtomicUnit=on
      settings: PermitHierarchicalResolution=ParametersOnly
  Memory : Memory  InheritSampleTime=on
  Multiply : Product
  Switch : Switch  Criteria=u2 > Threshold
  Out1 : Outport
  wires:
  In1/1 -> Multiply/2
  Multiply/1 -> Switch/3
  Constant1/1 -> Multiply/1
  Memory/1 -> Switch/2
  Switch/1 -> MATLAB Function/1(u), Out1/1, Memory/1
  Constant2/1 -> Switch/1

== system Citation_2015a/button2toggle 1/Triggered Subsystem ==
  In1 : Inport
  Trigger : TriggerPort
  Out1 : Outport
  wires:
  In1/1 -> Out1/1

== system Citation_2015a/Aero Forces & Moments /Aerodynamic Moment Components/Cl ==
  note: (q*r*(Izz-Iyy)*)+(pdot*Ixx)-(Ixz*(pq+rdot))
  model output : Inport
  Dynamic Pressure : Inport  Port=2
  Demux : Demux  Outputs=[1 1 1 9 1 1 1 22]
  Demux1 : Demux  Outputs=[4 1 1 1 1]
  Divide : Product  Inputs=*/
  Gain : Gain  Gain=span
  "Ixz*(pq+rdot) " : Product
  Sum : Sum  Inputs=|-+
  Sum1 : Sum  Inputs=|++
  Sum2 : Sum  Inputs=|-++
  Terminator{,1..2,6} (4 alike) : Terminator
  massinit : Constant  Value=massinit
  "pdot*Ixx " : Product
  pq : Product
  q*r*(Izz-Iyy) : Product  Inputs=3
  Cl : Outport
  wires:
  Demux/4 -> Terminator/1
  Demux/2 -> q*r*(Izz-Iyy)/1, pq/2  "q"
  Demux/5 -> "pdot*Ixx "/1  "pdot"
  massinit/1 -> Demux1/1
  Demux/1 -> pq/1  "p"
  Demux/8 -> Terminator1/1
  Demux1/2 -> "pdot*Ixx "/2  "Ixx"
  Demux/6 -> Terminator6/1  "qdot"
  Demux1/1 -> Terminator2/1
  model output/1 -> Demux/1
  Demux1/5 -> "Ixz*(pq+rdot) "/2  "Ixz"
  Demux/7 -> Sum1/2  "rdot"
  Demux/3 -> q*r*(Izz-Iyy)/2  "r"
  Demux1/3 -> Sum/1  "Iyy"
  Demux1/4 -> Sum/2  "Izz"
  Sum/1 -> q*r*(Izz-Iyy)/3
  pq/1 -> Sum1/1
  Sum1/1 -> "Ixz*(pq+rdot) "/1
  "Ixz*(pq+rdot) "/1 -> Sum2/1
  q*r*(Izz-Iyy)/1 -> Sum2/2
  "pdot*Ixx "/1 -> Sum2/3
  Dynamic Pressure/1 -> Gain/1
  Sum2/1 -> Divide/1
  Gain/1 -> Divide/2
  Divide/1 -> Cl/1

== system Citation_2015a/Aero Forces & Moments /Aerodynamic Moment Components/Cm ==
  "model output " : Inport
  Dynamic Pressure : Inport  Port=2
  Constant : Constant  Value=massinit
  Demux2 : Demux  Outputs=[1 1 1 9 1 1 1 22]
  Demux3 : Demux  Outputs=[4 1 1 1 1]
  Divide : Product  Inputs=*/
  Gain : Gain  Gain=chord
  Product{1,3..5} (4 alike) : Product
  Product2 : Product  Inputs=3
  Sum : Sum  Inputs=|+++
  Sum1 : Sum  Inputs=|+-
  Sum2 : Sum  Inputs=|+-
  Terminator{1..6} (6 alike) : Terminator
  Cm : Outport
  wires:
  Demux3/4 -> Sum1/2  "Izz"
  Demux2/8 -> Terminator4/1
  Demux3/5 -> Product5/2  "Ixz"
  Demux2/7 -> Terminator6/1  "rdot"
  Demux2/1 -> Product3/2, Product3/1, Product2/1  "p"
  Demux2/6 -> Product1/1  "qdot"
  Demux3/2 -> Sum1/1  "Ixx"
  Demux2/4 -> Terminator3/1
  Demux3/1 -> Terminator5/1
  Demux2/5 -> Terminator2/1  "pdot"
  Demux3/3 -> Product1/2  "Iyy"
  "model output "/1 -> Demux2/1
  Constant/1 -> Demux3/1
  Sum/1 -> Divide/1
  Divide/1 -> Cm/1
  Product1/1 -> Sum/2  "qdot*Iyy"
  Sum1/1 -> Product2/3
  Demux2/2 -> Terminator1/1  "q"
  Demux2/3 -> Product4/2, Product4/1, Product2/2  "r"
  Product2/1 -> Sum/1  "rp*(Ixx-Izz)"
  Product3/1 -> Sum2/1  "p^2"
  Product4/1 -> Sum2/2  "r^2"
  Sum2/1 -> Product5/1
  Product5/1 -> Sum/3  "(p^2 - r^2)*(Ixz)"
  Gain/1 -> Divide/2
  Dynamic Pressure/1 -> Gain/1

== system Citation_2015a/Aero Forces & Moments /Aerodynamic Moment Components/Cn ==
  model output : Inport
  Dynamic Pressure : Inport  Port=2
  Constant : Constant  Value=massinit
  Demux2 : Demux  Outputs=[1 1 1 9 1 1 1 22]
  Demux3 : Demux  Outputs=[4 1 1 1 1]
  Divide : Product  Inputs=*/
  Gain : Gain  Gain=span
  Product1 : Product
  Product2 : Product  Inputs=3
  Product3 : Product
  Product4 : Product
  Sum : Sum  Inputs=+++
  Sum1 : Sum  Inputs=|-+
  Sum2 : Sum  Inputs=|+-
  Terminator{1,3..5} (4 alike) : Terminator
  Cn : Outport
  wires:
  Demux3/4 -> Product1/2  "Izz"
  Demux2/8 -> Terminator4/1
  Demux3/5 -> Product3/2  "Ixz"
  Demux2/2 -> Product4/1, Product2/2  "q"
  Demux2/7 -> Product1/1  "rdot"
  Demux2/6 -> Terminator1/1  "qdot"
  Demux3/2 -> Sum1/1  "Ixx"
  Demux2/4 -> Terminator3/1
  Demux3/1 -> Terminator5/1
  Demux2/5 -> Sum2/2  "pdot"
  Demux3/3 -> Sum1/2  "Iyy"
  model output/1 -> Demux2/1
  Constant/1 -> Demux3/1
  Dynamic Pressure/1 -> Gain/1
  Sum/1 -> Divide/1  "rdot*Izz+pq*(Iyy-Ixx)+(qr-pdot)*Ixz"
  Product1/1 -> Sum/2  "rdot*Izz"
  Demux2/1 -> Product2/1  "p"
  Demux2/3 -> Product4/2  "r"
  Sum1/1 -> Product2/3
  Product2/1 -> Sum/1  "p*q*(Iyy-Ixx)"
  Product3/1 -> Sum/3  "Ixz*(qr-pdot)"
  Product4/1 -> Sum2/1
  Sum2/1 -> Product3/1
  Divide/1 -> Cn/1
  Gain/1 -> Divide/2  "0.5*rho*V^2*S*b"

== system Citation_2015a/Aerodynamic Parameter Estimation/Failure monitor system /Send message ==
  Trigger : TriggerPort
  MATLAB Function : MATLAB Function  TreatAsAtomicUnit=on
      settings: PermitHierarchicalResolution=ParametersOnly

== system Citation_2015a/Aerodynamic Parameter Estimation/Statistics 2/Auto_correlation ==
  delta_window : Inport
  kgap : Inport  Port=2
  Memory3 : Memory
  Memory4 : Memory
  autocorrelation : MATLAB Function  TreatAsAtomicUnit=on
      settings: PermitHierarchicalResolution=ParametersOnly
  PI_kgap : Outport
  PI_kgap_avg : Outport  Port=2
  wires:
  kgap/1 -> autocorrelation/2(kgap)
  autocorrelation/3(counter) -> Memory4/1
  Memory4/1 -> autocorrelation/4("counter ")
  autocorrelation/1(PI_kgap) -> PI_kgap/1
  autocorrelation/2(kgap_avg) -> Memory3/1, PI_kgap_avg/1
  Memory3/1 -> autocorrelation/3("kgap_avg ")
  delta_window/1 -> autocorrelation/1(delta)

== system Citation_2015a/Aerodynamic Parameter Estimation/Statistics 2/variance ==
  delta : Inport
  MATLAB Function : MATLAB Function  TreatAsAtomicUnit=on
      settings: PermitHierarchicalResolution=ParametersOnly
  Memory : Memory
  Memory1 : Memory
  Memory2 : Memory  X0=[0, 0]
  variance : Outport
  sigma_avg : Outport  Port=2
  wires:
  Memory1/1 -> MATLAB Function/2("delta_avg ")
  MATLAB Function/4(sigma_avg) -> sigma_avg/1, Memory2/1
  Memory2/1 -> MATLAB Function/4("sigma_avg ")
  MATLAB Function/2(delta_avg) -> Memory1/1  "average"
  Memory/1 -> MATLAB Function/3("counter ")
  MATLAB Function/1(var) -> variance/1
  MATLAB Function/3(counter) -> Memory/1
  delta/1 -> MATLAB Function/1(delta)

== system Citation_2015a/Aerodynamic Parameter Estimation/Statistics 3/Auto_correlation ==
  delta_window : Inport
  kgap : Inport  Port=2
  Memory3 : Memory
  Memory4 : Memory
  autocorrelation : MATLAB Function  TreatAsAtomicUnit=on
      settings: PermitHierarchicalResolution=ParametersOnly
  PI_kgap : Outport
  PI_kgap_avg : Outport  Port=2
  wires:
  delta_window/1 -> autocorrelation/1(delta)
  Memory3/1 -> autocorrelation/3("kgap_avg ")
  autocorrelation/2(kgap_avg) -> PI_kgap_avg/1, Memory3/1
  autocorrelation/1(PI_kgap) -> PI_kgap/1
  Memory4/1 -> autocorrelation/4("counter ")
  autocorrelation/3(counter) -> Memory4/1
  kgap/1 -> autocorrelation/2(kgap)

== system Citation_2015a/Aerodynamic Parameter Estimation/Statistics 3/variance ==
  delta : Inport
  MATLAB Function : MATLAB Function  TreatAsAtomicUnit=on
      settings: PermitHierarchicalResolution=ParametersOnly
  Memory : Memory
  Memory1 : Memory
  Memory2 : Memory  X0=[0, 0]
  variance : Outport
  sigma_avg : Outport  Port=2
  wires:
  delta/1 -> MATLAB Function/1(delta)
  MATLAB Function/3(counter) -> Memory/1
  MATLAB Function/1(var) -> variance/1
  Memory/1 -> MATLAB Function/3("counter ")
  MATLAB Function/2(delta_avg) -> Memory1/1  "average"
  Memory2/1 -> MATLAB Function/4("sigma_avg ")
  MATLAB Function/4(sigma_avg) -> Memory2/1, sigma_avg/1
  Memory1/1 -> MATLAB Function/2("delta_avg ")

== system Citation_2015a/Aerodynamic Parameter Estimation/Statistics 4/Auto_correlation ==
  delta_window : Inport
  kgap : Inport  Port=2
  Memory3 : Memory
  Memory4 : Memory
  autocorrelation : MATLAB Function  TreatAsAtomicUnit=on
      settings: PermitHierarchicalResolution=ParametersOnly
  PI_kgap : Outport
  PI_kgap_avg : Outport  Port=2
  wires:
  kgap/1 -> autocorrelation/2(kgap)
  autocorrelation/3(counter) -> Memory4/1
  Memory4/1 -> autocorrelation/4("counter ")
  autocorrelation/1(PI_kgap) -> PI_kgap/1
  autocorrelation/2(kgap_avg) -> Memory3/1, PI_kgap_avg/1
  Memory3/1 -> autocorrelation/3("kgap_avg ")
  delta_window/1 -> autocorrelation/1(delta)

== system Citation_2015a/Aerodynamic Parameter Estimation/Statistics 4/variance ==
  delta : Inport
  MATLAB Function : MATLAB Function  TreatAsAtomicUnit=on
      settings: PermitHierarchicalResolution=ParametersOnly
  Memory : Memory
  Memory1 : Memory
  Memory2 : Memory  X0=[0, 0]
  variance : Outport
  sigma_avg : Outport  Port=2
  wires:
  Memory1/1 -> MATLAB Function/2("delta_avg ")
  MATLAB Function/4(sigma_avg) -> sigma_avg/1, Memory2/1
  Memory2/1 -> MATLAB Function/4("sigma_avg ")
  MATLAB Function/2(delta_avg) -> Memory1/1  "average"
  Memory/1 -> MATLAB Function/3("counter ")
  MATLAB Function/1(var) -> variance/1
  MATLAB Function/3(counter) -> Memory/1
  delta/1 -> MATLAB Function/1(delta)

== system Citation_2015a/Aerodynamic Parameter Estimation/alternative failure monitor system/Auto_correlation ==
  delta_window : Inport
  kgap : Inport  Port=2
  Memory3 : Memory
  Memory4 : Memory
  autocorrelation : MATLAB Function  TreatAsAtomicUnit=on
      settings: PermitHierarchicalResolution=ParametersOnly
  PI_kgap : Outport
  PI_kgap_avg : Outport  Port=2
  wires:
  delta_window/1 -> autocorrelation/1(delta)
  Memory3/1 -> autocorrelation/3("kgap_avg ")
  autocorrelation/2(kgap_avg) -> PI_kgap_avg/1, Memory3/1
  autocorrelation/1(PI_kgap) -> PI_kgap/1
  Memory4/1 -> autocorrelation/4("counter ")
  autocorrelation/3(counter) -> Memory4/1
  kgap/1 -> autocorrelation/2(kgap)

== system Citation_2015a/Aerodynamic Parameter Estimation/alternative failure monitor system/Send diagnostic message ==
  In1 : Inport
  Trigger : TriggerPort  TriggerType=either
  MATLAB Function : MATLAB Function  TreatAsAtomicUnit=on
      settings: PermitHierarchicalResolution=ParametersOnly
  wires:
  In1/1 -> MATLAB Function/1(u)

== system Citation_2015a/Aerodynamic Parameter Estimation/alternative failure monitor system/Slider ==

== system Citation_2015a/Aerodynamic Parameter Estimation/alternative failure monitor system/variance ==
  delta : Inport
  MATLAB Function : MATLAB Function  TreatAsAtomicUnit=on
      settings: PermitHierarchicalResolution=ParametersOnly
  Memory : Memory
  Memory1 : Memory
  Memory2 : Memory  X0=[0, 0]
  variance : Outport
  sigma_avg : Outport  Port=2
  wires:
  delta/1 -> MATLAB Function/1(delta)
  MATLAB Function/3(counter) -> Memory/1
  MATLAB Function/1(var) -> variance/1
  Memory/1 -> MATLAB Function/3("counter ")
  MATLAB Function/2(delta_avg) -> Memory1/1  "average"
  Memory2/1 -> MATLAB Function/4("sigma_avg ")
  MATLAB Function/4(sigma_avg) -> Memory2/1, sigma_avg/1
  Memory1/1 -> MATLAB Function/2("delta_avg ")

== system Citation_2015a/Cessna Citation 500/Actuators/Subsystem ==
  failure toggle : Inport
  Aileron : Inport  Port=2
  Display2 : Display
  Fcn : Fcn  Expr=u>=16
  Memory : Memory  InheritSampleTime=on
  Multiply : Product
  Multiply1 : Product
  Saturation : Saturate  UpperLimit=1
  Sum1 : Sum  Inputs=|++
  deg2rad1 : Gain  Gain=180/pi
  switch signal : Outport
  wires:
  Aileron/1 -> deg2rad1/1
  Fcn/1 -> Multiply/1
  deg2rad1/1 -> Fcn/1
  Saturation/1 -> Multiply1/1
  failure toggle/1 -> Multiply1/2, Multiply/2
  Memory/1 -> Sum1/2
  Multiply1/1 -> switch signal/1, Memory/1, Display2/1
  Sum1/1 -> Saturation/1
  Multiply/1 -> Sum1/1

== system Citation_2015a/Cessna Citation 500/Actuators/da ==
  In : Inport
  Gain : Gain  Gain=13  SaturateOnIntegerOverflow=on  OutDataTypeStr=Inherit: Same as input  ParamDataTypeStr=Inherit: Same as input
  Integrator : Integrator  InitialCondition=u0(2)
  Sum : Sum  Inputs=|+-  SaturateOnIntegerOverflow=on
  Out : Outport
  wires:
  Integrator/1 -> Out/1, Sum/2
  In/1 -> Sum/1
  Sum/1 -> Gain/1
  Gain/1 -> Integrator/1

== system Citation_2015a/Cessna Citation 500/Actuators/da2 ==
  In : Inport
  Gain : Gain  Gain=13  SaturateOnIntegerOverflow=on  OutDataTypeStr=Inherit: Same as input  ParamDataTypeStr=Inherit: Same as input
  Integrator : Integrator  InitialCondition=u0(2)
  Sum : Sum  Inputs=|+-  SaturateOnIntegerOverflow=on
  Out : Outport
  wires:
  Integrator/1 -> Out/1, Sum/2
  In/1 -> Sum/1
  Sum/1 -> Gain/1
  Gain/1 -> Integrator/1

== system Citation_2015a/Cessna Citation 500/Actuators/de ==
  In : Inport
  Gain : Gain  Gain=13  SaturateOnIntegerOverflow=on  OutDataTypeStr=Inherit: Same as input  ParamDataTypeStr=Inherit: Same as input
  Integrator : Integrator  InitialCondition=u0(1)
  Sum : Sum  Inputs=|+-  SaturateOnIntegerOverflow=on
  Out : Outport
  wires:
  Integrator/1 -> Out/1, Sum/2
  In/1 -> Sum/1
  Sum/1 -> Gain/1
  Gain/1 -> Integrator/1

== system Citation_2015a/Cessna Citation 500/Actuators/dr ==
  In : Inport
  Gain : Gain  Gain=13  SaturateOnIntegerOverflow=on  OutDataTypeStr=Inherit: Same as input  ParamDataTypeStr=Inherit: Same as input
  Integrator : Integrator  InitialCondition=u0(3)
  Sum : Sum  Inputs=|+-  SaturateOnIntegerOverflow=on
  Out : Outport
  wires:
  Integrator/1 -> Out/1, Sum/2
  In/1 -> Sum/1
  Sum/1 -> Gain/1
  Gain/1 -> Integrator/1

== system Citation_2015a/Cessna Citation 500/Actuators/flaps ==
  In : Inport
  Gain : Gain  Gain=0.9  SaturateOnIntegerOverflow=on  OutDataTypeStr=Inherit: Same as input  ParamDataTypeStr=Inherit: Same as input
  Integrator : Integrator  InitialCondition=u0(7)
  Sum : Sum  Inputs=|+-  SaturateOnIntegerOverflow=on
  Out : Outport
  wires:
  Integrator/1 -> Out/1, Sum/2
  In/1 -> Sum/1
  Sum/1 -> Gain/1
  Gain/1 -> Integrator/1

== system Citation_2015a/Cessna Citation 500/Actuators/gear ==
  In : Inport
  Gain : Gain  Gain=0.6  SaturateOnIntegerOverflow=on  OutDataTypeStr=Inherit: Same as input  ParamDataTypeStr=Inherit: Same as input
  Integrator : Integrator  InitialCondition=u0(8)
  Sum : Sum  Inputs=|+-  SaturateOnIntegerOverflow=on
  Out : Outport
  wires:
  Integrator/1 -> Out/1, Sum/2
  In/1 -> Sum/1
  Sum/1 -> Gain/1
  Gain/1 -> Integrator/1
